simulink model "ammclib_gflib_pidp_s32k11x"  (Simulink 9.0)
settings: Solver=FixedStepDiscrete  StartTime=0.0  StopTime=5  FixedStep=0.001  RelTol=1e-3  EnableMultiTasking=on
InitFcn:
  | mbd_s32k_consistency_checks(bdroot(gcs));
undefined symbols (not defined in the file): LQFP, thumb
libraries: ammclib_bam_s32k11x x3, mbd_s32k1xx_ec_toolbox x2, simulink x1
Description:
  | This model tests the AMMCLIB GFLIB PI Recurent Form Controller blocks
  | 
  | Validation:
  | - Run the model in Simulation and check if the results look like the ones shown in the scope capture
  | - Open Freemaster (ammclib_gflib_pir_s32k11x.pmp) and compare the HW results against the Simulated ones
CloseFcn:
  | clear all;
settings Model: Creator=NXP MBDT Team  LastModifiedBy=nxf35172
settings DataIOCC: ExternalInput=off  InitialState=off  LimitDataPoints=on  SaveOutput=off  SignalLogging=off  SaveTime=off
settings OptimizationCC: DefaultParameterBehavior=Inlined  LifeSpan=1
settings DebuggingCC: SolverPrmCheckMsg=warning  InheritedTsInSrcMsg=none  SingleTaskRateTransMsg=error  ParameterPrecisionLossMsg=none  UnconnectedInputMsg=error  UnconnectedOutputMsg=error  UnconnectedLineMsg=error  AllowSymbolicDim=off  UnknownTsInhSupMsg=error  StateNameClashWarn=warning
settings HardwareCC: ProdLargestAtomicInteger=Long  ProdLargestAtomicFloat=Double  ProdEndianess=LittleEndian  ProdHWDeviceType=ARM Compatible->ARM Cortex
settings SFSimCC: MATLABDynamicMemAlloc=off
settings RTWCC: SystemTargetFile=mbd_s32k.tlc  MakeCommand=mbd_s32k_make_rtw COPY_MDLREF_INCLUDES=0  TemplateMakefile=mbd_s32k.tmf  Description=Model Based Design Toolbox S32K14x Code Generation Target
settings CodeAppCC: IgnoreCustomStorageClasses=off
settings STFCustomTargetCC: CombineOutputUpdateFcns=on  ERTCustomFileBanners=on  SupportContinuousTime=off  SupportNonInlinedSFcns=off  RemoveResetFunc=on  MATLABClassNameForMDSCustomization=Simulink.SoftwareTarget.ERTCustomization  GRTInterface=off  SystemTargetFile=mbd_s32k14.tlc
settings ERTTargetCC: MultiwordLength=2048  ParMdlRefBuildCompliant=off  CompOptLevelCompliant=off  ConcurrentExecutionCompliant=off  ModelStepFunctionPrototypeControlCompliant=off  CPPClassGenCompliant=off  UseToolchainInfoCompliant=off  InlinedParameterPlacement=NonHierarchical  ERTCustomFileTemplate=example_file_process.tlc  ConvertIfToSwitch=off  SuppressUnreachableDefaultCases=off  MaxIdInt32=FIRX_int32_T  MaxIdUint32=FIRX_uint32_T  MaxIdInt16=FIRX_int16_T  MaxIdUint16=FIRX_uint16_T  MaxIdInt8=FIRX_int8_T  MaxIdUint8=FIRX_uint8_T

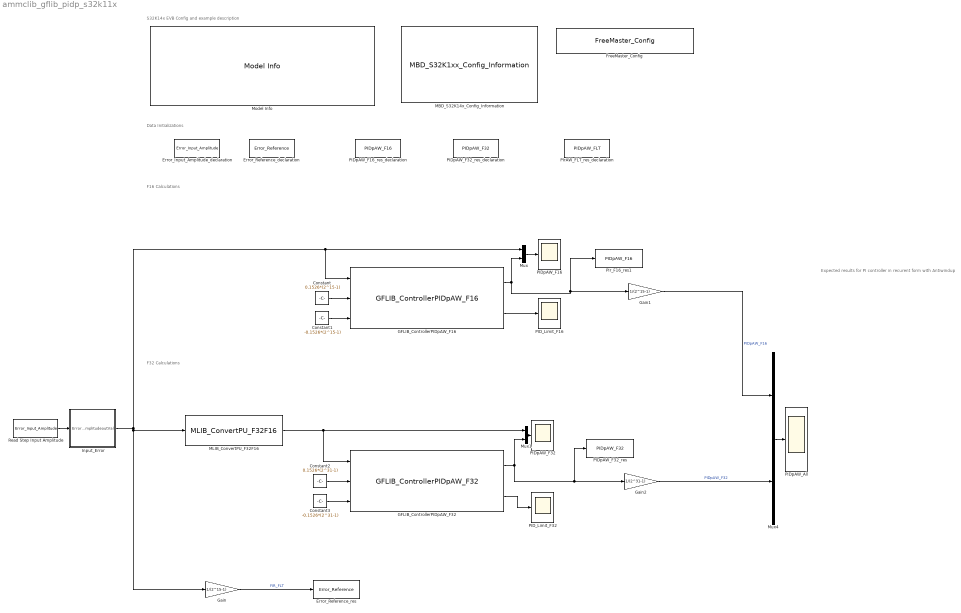
== system ammclib_gflib_pidp_s32k11x ==
  note: Expected results for PI controller in recurent form with Antiwindup
  note: S32K14x EVB Config and example description
  note: Data Initializations
  note: F16 Calculations
  note: F32 Calculations
  Constant : Constant  Value=0.1526*(2^15-1)  OutDataTypeStr=Inherit: Inherit via back propagation
  Constant1 : Constant  Value=-0.1526*(2^15-1)  OutDataTypeStr=Inherit: Inherit via back propagation
  Constant2 : Constant  Value=0.1526*(2^31-1)  OutDataTypeStr=Inherit: Inherit via back propagation
  Constant3 : Constant  Value=-0.1526*(2^31-1)  OutDataTypeStr=Inherit: Inherit via back propagation
  Error_Input_Amplitude_declaration : DataStoreMemory  Priority=1  DataStoreName=Error_Input_Amplitude  WriteAfterWriteMsg=warning  WriteAfterReadMsg=warning  InitialValue=8192  ShowAdditionalParam=off  OutMin=-32768  OutMax=32767  OutDataTypeStr=int16
  Error_Reference_declaration : DataStoreMemory  Priority=1  DataStoreName=Error_Reference  WriteAfterWriteMsg=warning  WriteAfterReadMsg=warning  ShowAdditionalParam=off  OutMin=-1  OutMax=1  OutDataTypeStr=single
  Error_Reference_res : DataStoreWrite  DataStoreName=Error_Reference
  FreeMaster_Config : mbd_s32k1xx_ec_toolbox/Utility Blocks/FreeMaster_Config  interface=LPUART0  baudrate=19200  rxd=PTB0: [LPUART0_RX | Receive]  txd=PTB1: [LPUART0_TX | Transmit]  mode=Short Interrupt  isr_prio=0  show_adv_opts=off  use_scope=on  max_scope_vars=8  use_recorder=on  max_rec_vars=8  rec_buff_size=1024  rec_timebase=0 milliseconds  comm_buffer_size_auto=on  comm_buffer_size=255  comm_rqueue_size_default=on  comm_rqueue_size=32
  GFLIB_ControllerPIDpAW_F16 : ammclib_bam_s32k11x/GFLIB/bam_f16/GFLIB_ControllerPIDpAW_F16  f16PropGain=0.006*(2^15-1)  s16PropGainShift=0  f16IntegGain=0.0006*(2^15-1)  s16IntegGainShift=0  f16DerivGain=0.001*(2^15-1)  s16DerivGainShift=0  f16FiltCoef=0.4*(2^15-1)
  GFLIB_ControllerPIDpAW_F32 : ammclib_bam_s32k11x/GFLIB/bam_f32/GFLIB_ControllerPIDpAW_F32  f32PropGain=0.006*(2^31-1)  s16PropGainShift=0  f32IntegGain=0.0006*(2^31-1)  s16IntegGainShift=0  f32DerivGain=0.001*(2^31-1)  s16DerivGainShift=0  f32FiltCoef=0.4*(2^31-1)
  Gain : Gain  Gain=1/(2^15-1)  OutDataTypeStr=Inherit: Inherit via back propagation
  Gain1 : Gain  Gain=1/(2^15-1)  ParamDataTypeStr=single
  Gain2 : Gain  Gain=1/(2^31-1)  ParamDataTypeStr=single
  Input_Error : Stateflow chart  TreatAsAtomicUnit=on
  MBD_S32K14x_Config_Information : mbd_s32k1xx_ec_toolbox/MBD_S32K1xx_Config_Information  Priority=0  mbdt_ver=0  disp_str=|  config_params=[]  mcu_target_name=S32K116  mcu_target_package=48-LQFP  mcu_target_sram_size=17KB  mcu_system_clock_freq=40  mcu_xtal_freq=External 40  mcu_steptick_timer=LPIT Channel 0  mcu_steptick_prio=0  ds_import_enable=on  target_compiler=GCC  target_memory=FLASH  gcc_target_compile_opts=-mcpu=cortex-m0plus -mthumb -O1 -g -gstrict-dwarf  gcc_target_assemble_opts=-mcpu=cortex-m0plus -mthumb -g  gcc_target_link_opts=-mcpu=cortex-m0plus -mthumb  gcc_target_default_lcf=on  gcc_target_user_lcf=S32K116_17_flash.ld  ghs_target_compile_opts=-mcpu=cortexm0plus -mthumb -fsoft -Ogeneral -Wundef -Wimplicit-int -Wshadow -Wtrigraphs --no_commons --gnu_asm -gnu99 -gdwarf-2 -G  ghs_target_assemble_opts=-mcpu=cortexm0plus -mthumb -fsoft --gnu_asm  ghs_target_link_opts=-mcpu=cortexm0plus -mthumb -fsoft  ghs_target_default_lcf=off  ghs_target_user_lcf=S32K116_17_flash.ld  iar_target_compile_opts=--thumb -Ol -e --debug --dlib_config normal  iar_target_assemble_opts=--thumb  iar_target_link_opts=--no_exceptions --vfe --inline  iar_target_default_lcf=off  iar_target_user_lcf=S32K116_17_flash.icf  pil_download_enable=off  rbl_download_enable=on  rbl_start_delay=5000000  rbl_download_interface=OpenSDA  rbl_restart_request=off  rbl_com_port=Custom  rbl_com_port_custom=COM1  pil_download_rate=57600  pil_opensda_drive=Custom  pil_opensda_drive_custom=D  pil_uart_instance=0  pil_uart_rx=PTA2: [LPUART0_RX | Receive]  pil_uart_tx=PTA3: [LPUART0_TX | Transmit]  FTM_PWM_PcrCheckEnDis=on  FTM_Input_Edge_Inputs_PcrCheckEnDis=on  FTM_Dual_Edge_Inputs_PcrCheckEnDis=on  FTM_Quadrature_Inputs_PcrCheckEnDis=on  FTM_Hall_Sensor_Inputs_PcrCheckEnDis=on  LPTMR_PcrCheckEnDis=on  PIT_PcrCheckEnDis=on  RTC_PcrCheckEnDis=on  FlexCAN_PcrCheckEnDis=on  LIN_PcrCheckEnDis=on  FlexIO_PcrCheckEnDis=on  LPI2C_PcrCheckEnDis=on  LPSPI_PcrCheckEnDis=on  LPUART_PcrCheckEnDis=on  CMP_PcrCheckEnDis=on  GPIO_OutputPcrCheckEnDis=on  GPIO_InputPcrCheckEnDis=on  SBC_PcrCheckEnDis=on  AMMCLIB_PcrCheckEnDis=on  FM_PcrCheckEnDis=on  Profile_PcrCheckEnDis=on  ConfigParams_PcrCheckEnDis=on  ModelRef_PcrCheckEnDis=on  PDB0_PcrCheckEnDis=on  CSEc_PcrCheckEnDis=on  eDMA_PcrCheckEnDis=on  ADC_PcrCheckEnDis=on  WDOG_PcrCheckEnDis=on
      | Target : S32K142-16KB_SRAM
      | Package : 100-pin
      | System clock : 80 MHz
      | XTAL clock : External 8 MHz
      | Compiler : GCC
      | Target Type : FLASH
      | Download Code after build : (OpenSDA: E)
      | Step Tick Interrupt Priority : 15
  MLIB_ConvertPU_F32F16 : ammclib_bam_s32k11x/MLIB/bam_f32/MLIB_ConvertPU_F32F16
  Model Info : simulink/Model-Wide Utilities/Model Info  Frame=off  DisplayStringWithTags=|  HorizontalTextAlignment=Left  LeftAlignmentValue=0.02
      | Model Name: %<ModelName>
      | 
      | Description: %<Description>
  Mux : Mux  Inputs=2
  Mux1 : Mux  Inputs=2
  Mux4 : Mux  Inputs=2
  PID_Limit_F16 : Scope
  PID_Limit_F32 : Scope
  PIDpAW_All : Scope
  PIDpAW_F16 : Scope
  PIDpAW_F16_res_declaration : DataStoreMemory  Priority=2  DataStoreName=PIDpAW_F16  ReadBeforeWriteMsg=warning  WriteAfterWriteMsg=warning  WriteAfterReadMsg=warning  ShowAdditionalParam=off  OutDataTypeStr=int16
  PIDpAW_F32 : Scope
  PIDpAW_F32_res : DataStoreWrite  DataStoreName=PIDpAW_F32
  PIDpAW_F32_res_declaration : DataStoreMemory  Priority=2  DataStoreName=PIDpAW_F32  ReadBeforeWriteMsg=warning  WriteAfterWriteMsg=warning  WriteAfterReadMsg=warning  ShowAdditionalParam=off  OutDataTypeStr=int32
  PIrAW_FLT_res_declaration : DataStoreMemory  Priority=2  DataStoreName=PIDpAW_FLT  ReadBeforeWriteMsg=warning  WriteAfterWriteMsg=warning  WriteAfterReadMsg=warning  ShowAdditionalParam=off  OutDataTypeStr=single
  PIr_F16_res1 : DataStoreWrite  DataStoreName=PIDpAW_F16
  Read Step Input Amplitude : DataStoreRead  DataStoreName=Error_Input_Amplitude
  wires:
  Mux/1 -> PIDpAW_F16/1
  Read Step Input Amplitude/1 -> Input_Error/1(Error_Input_Amplitude)
  Gain/1 -> Error_Reference_res/1  "FIR_FLT"
  Constant/1 -> GFLIB_ControllerPIDpAW_F16/2
  Constant1/1 -> GFLIB_ControllerPIDpAW_F16/3
  Gain1/1 -> Mux4/1  "PIDpAW_F16"
  GFLIB_ControllerPIDpAW_F32/1 -> Mux1/2, Gain2/1, PIDpAW_F32_res/1
  Mux1/1 -> PIDpAW_F32/1
  MLIB_ConvertPU_F32F16/1 -> GFLIB_ControllerPIDpAW_F32/1, Mux1/1
  Constant2/1 -> GFLIB_ControllerPIDpAW_F32/2
  Constant3/1 -> GFLIB_ControllerPIDpAW_F32/3
  Gain2/1 -> Mux4/2  "PIDpAW_F32"
  Mux4/1 -> PIDpAW_All/1
  GFLIB_ControllerPIDpAW_F16/2 -> PID_Limit_F16/1
  GFLIB_ControllerPIDpAW_F32/2 -> PID_Limit_F32/1
  Input_Error/1(outVal) -> GFLIB_ControllerPIDpAW_F16/1, Mux/1, Gain/1, MLIB_ConvertPU_F32F16/1
  GFLIB_ControllerPIDpAW_F16/1 -> Mux/2, Gain1/1, PIr_F16_res1/1

== stateflow chart Input_Error ==
  settings: executeAtInitialization=1
  state A
    du:
    outVal = Error_Input_Amplitude;
    cntr=cntr+1;
  state A1
    du:
    outVal = -Error_Input_Amplitude;
    cntr=cntr-1;
  (default) -> A : {cntr=0;}
  A1 -> A : [cntr < 2]
  A -> A1 : [cntr > 1000]
  data: cntr local uint32 [0..12] =0; outVal output int16; Error_Input_Amplitude input int16
